simulink model "Test_T_Matrix_VSC"  (R2024a)
settings: Solver=ode2  StartTime=0.0  StopTime=T_end  RelTol=1e-3  EnableMultiTasking=on
values from neighbouring files (symbols this model uses):
  Ts = 5e-6    (= 5e-06)    [Generate_T_Matrix.m]    (also in Test_T_Matrix.m)
undefined symbols (not defined in the file or in its folder): level
libraries: spsabctodq0Lib x5, slpidlib x4, powerlib_extras x3, spsThreePhaseVIMeasurementLib x3, spsThreePhaseSeriesRLCBranchLib x2, simulink_extras x2, spsThreePhaseProgrammableVoltageSourceLib x1, spsGroundLib x1, spsThreePhaseFaultLib x1, spsDCVoltageSourceLib x1, spsUniversalBridgeLib x1, spsdq0toabcLib x1
settings Model: Creator=GAO_CX  LastModifiedBy=GAO_CX
settings DataIOCC: SaveOutput=off  SignalLogging=off  DSMLogging=off  SaveTime=off  ReturnWorkspaceOutputs=off

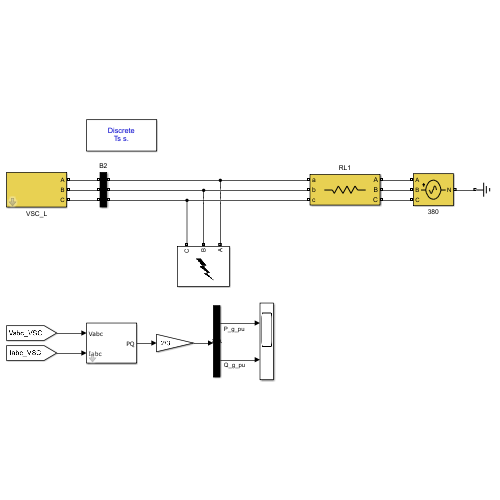
[thumbnail: Simulink's stored preview of the top-level diagram]
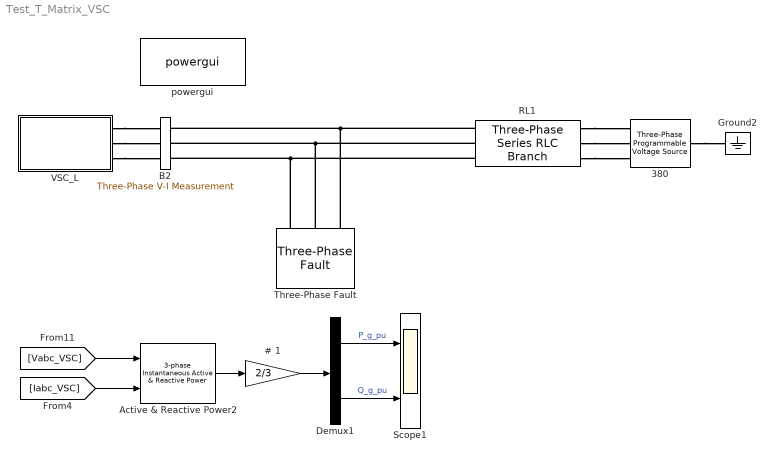
== system Test_T_Matrix_VSC ==
  # 1 : Gain  Gain=2/3  SaturateOnIntegerOverflow=on  OutDataTypeStr=Inherit: Same as input  ParamDataTypeStr=Inherit: Same as input
  380 : spsThreePhaseProgrammableVoltageSourceLib/Three-Phase Programmable Voltage Source  PositiveSequence=[380 0 50]  VariationEntity=None  VariationType=Step  VariationTypeAlt=Step  VariationStep=0.2  VariationRate=10  VariationMagnitude=0.3  VariationFrequency=2  VariationTiming=[20 20.05]  VariationPhaseA=off  Amplitudes=[1 0.5 1]  TimeValues=[0 20 20.3]  HarmonicGeneration=off  HarmonicA=[1 -0.1 0 2]  HarmonicB=[2 0.15 35 2]*0  Timing="[0.1  2]"  BusType=PQ  Pref=0  Qref=0  Qmin=-inf  Qmax=inf
  Active & Reactive Power2 : powerlib_extras/Measurements/3-phase  Instantaneous  Active & Reactive Power
  B2 : spsThreePhaseVIMeasurementLib/Three-Phase V-I Measurement  VoltageMeasurement=phase-to-ground  SetLabelV=on  LabelV=Vabc_VSC  Vpu=on  VpuLL=off  CurrentMeasurement=yes  SetLabelI=on  LabelI=Iabc_VSC  Ipu=on  Pbase=1e6  Vbase=380  OutputType=Complex  PhasorSimulation=off  PSBequivalent=0
  Demux1 : Demux  Outputs=2
      settings: DisplayOption=none
  Ground2 : spsGroundLib/Ground  LConnTagsString=a
  RL1 : spsThreePhaseSeriesRLCBranchLib/Three-Phase Series RLC Branch  LConnTagsString=A|B|C  RConnTagsString=A|B|C  BranchType=R  Resistance=0.01  Inductance=4e-6  Capacitance=1.0  Measurements=None
  Scope1 : Scope  NumInputPorts=2
  Three-Phase Fault : spsThreePhaseFaultLib/Three-Phase Fault  InitialStates=0  FaultA=on  FaultB=off  FaultC=off  GroundFault=on  SwitchTimes=[0.1 0.15]  External=off  SwitchStatus=NaN  FaultResistance=1e-6  GroundResistance=1e-9  SnubberResistance=inf  SnubberCapacitance=inf  Measurements=None
  VSC_L : Subsystem  mask{P_rated=1e6, Vac_rated=380, Vdc_rated=1200, f_rated=50, Pref=1.0, Qref=0, Rf1_pu=1e-3, Lf1_pu=0.5, KP_PLL=5, KI_PLL=100, KP_ig=5, KI_ig=10, KP_P=0.2, KI_P=100}
      mask prompts: P_rated "Rated Power (W)"; Vac_rated "Rated AC voltage (V)"; Vdc_rated "Rated DC voltage (V)"; f_rated "Rated grid frequency"; Rf1_pu "Filter resistor Rf1 (pu)"; Lf1_pu "Filter inductor Lf1 (pu)"; KP_PLL "P of PLL"; KI_PLL "I of PLL"; KP_ig "P of current PI  controller"; KI_ig "I of current PI  controller"; KP_P "P of power PI  controller"; KI_P "I of power PI  controller"
      mask init:
      | Z_rated=Vac_rated*Vac_rated/P_rated;
      | % transformer to pu
      | wg_rated=2*pi*f_rated;
      | Lg_rated=Z_rated/wg_rated;
      | Cg_rated=1/Z_rated/wg_rated;
      | 
      | Rf1=Z_rated*Rf1_pu;
      | Lf1=Lg_rated*Lf1_pu;
      mask DialogControl Basic_Parameters Prompt: Basic Parameters
      mask DialogControl GSC Prompt: GSC Parameters
  powergui : spspowerguiLib/powergui  SimulationMode=Discrete  SampleTime=Ts  frequency=50  Iterations=50  frequencyindice=0  Pbase=100e6  ErrMax=1e-4  UnitsV=kV  UnitsW=MW  buscounter=6  FunctionMessages=off  echomessages=off  EnableUseOfTLC=off  CurrentSourceSwitches=off  DisableSnubberDevices=off  DisableRonSwitches=off  DisableVfSwitches=off  DisplayEquations=off  AutomaticDiscreteSolvers=off  SolverType=Tustin  Interpol=off  ExternalGateDelay=off  methode=off  Ts=0  x0status=blocks  SPID=off  SwTol=0  HookPort=off  NonlinearTolerance=1e-4  nMaxIteration=100  ContinueOnMaxIteration=off  RestoreLinks=warning  ResistiveCurrentMeasurement=off  Frange=[0:2:500]  Ylog=off  Xlog=on  ShowGrid=off  save=off  variable=ZData  structure=0  ZoomFFT=on  StartTime=0.0  cycles=1  DisplayStyle=1  fundamental=60  FreqAxis=off  MaxFrequency=1000  frequencyindicesteady=1  RmsSteady=1  display=off
  wires:
  Demux1/1 -> Scope1/1  "P_g_pu"
  Demux1/2 -> Scope1/2  "Q_g_pu"
  Active & Reactive Power2/1 -> # 1/1
  # 1/1 -> Demux1/1
  [Vabc_VSC] -> Active & Reactive Power2/1
  [Iabc_VSC] -> Active & Reactive Power2/2
  connections:
  RL1/RConn2 -- Three-Phase Fault/LConn2 -- B2/RConn2
  VSC_L/LConn3 -- B2/LConn3
  RL1/LConn1 -- 380/RConn1
  380/LConn1 -- Ground2/LConn1
  VSC_L/LConn1 -- B2/LConn1
  RL1/LConn3 -- 380/RConn3
  VSC_L/LConn2 -- B2/LConn2
  RL1/LConn2 -- 380/RConn2
  RL1/RConn3 -- B2/RConn3 -- Three-Phase Fault/LConn3
  RL1/RConn1 -- Three-Phase Fault/LConn1 -- B2/RConn1

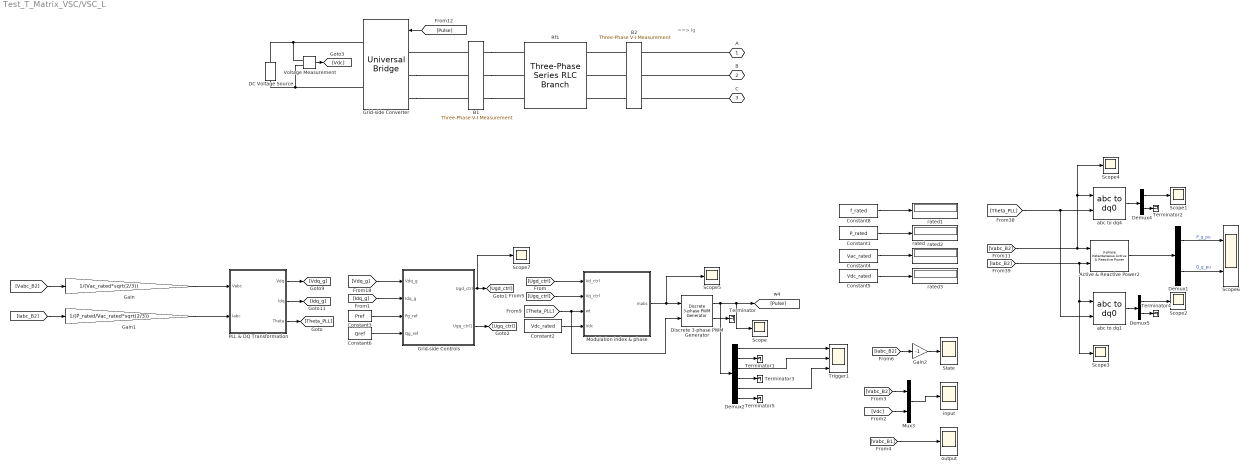
== system Test_T_Matrix_VSC/VSC_L ==
  note: ==> Ig
  Active & Reactive Power2 : powerlib_extras/Measurements/3-phase  Instantaneous  Active & Reactive Power
  B1 : spsThreePhaseVIMeasurementLib/Three-Phase V-I Measurement  VoltageMeasurement=phase-to-ground  SetLabelV=on  LabelV=Vabc_B1  Vpu=off  VpuLL=off  CurrentMeasurement=no  SetLabelI=off  LabelI=Iabc_B1  Ipu=off  Pbase=P_rated  Vbase=Vac_rated  OutputType=Complex  PhasorSimulation=off  PSBequivalent=0
  B2 : spsThreePhaseVIMeasurementLib/Three-Phase V-I Measurement  VoltageMeasurement=phase-to-ground  SetLabelV=on  LabelV=Vabc_B2  Vpu=off  VpuLL=off  CurrentMeasurement=yes  SetLabelI=on  LabelI=Iabc_B2  Ipu=off  Pbase=P_rated  Vbase=Vac_rated  OutputType=Complex  PhasorSimulation=off  PSBequivalent=0
  Constant1 : Constant  Value=P_rated
  Constant2 : Constant  Value=Vdc_rated
  Constant3 : Constant  Value=Pref
  Constant4 : Constant  Value=Vac_rated
  Constant5 : Constant  Value=Vdc_rated
  Constant6 : Constant  Value=Qref
  Constant8 : Constant  Value=f_rated
  DC Voltage Source : spsDCVoltageSourceLib/DC Voltage Source  Amplitude=Vdc_rated  Measurements=None
  Demux1 : Demux  Outputs=2
      settings: DisplayOption=none
  Demux2 : Demux  Outputs=6
      settings: DisplayOption=none
  Demux4 : Demux  Outputs=[2 1]
      settings: DisplayOption=none
  Demux5 : Demux  Outputs=[2 1]
      settings: DisplayOption=none
  Discrete 3-phase PWM Generator : powerlib_extras/Discrete  Control Blocks/Discrete 3-phase PWM Generator  ModulatorType=2-level  ModulatorMode=Synchronized  nF=100  Fc=2700  ModulatingSignals=off  m=0.2  Freq=60  Phase=0  Ts=Ts
  Gain : Gain  Gain=1/(Vac_rated*sqrt(2/3))
  Gain1 : Gain  Gain=1/(P_rated/Vac_rated*sqrt(2/3))
  Gain2 : Gain  Gain=-1
  Grid-side Converter : spsUniversalBridgeLib/Universal Bridge  Arms=3  SnubberResistance=1e6  SnubberCapacitance=inf  Device=IGBT / Diodes  Ron=0.01  Lon=0  ForwardVoltages="[  0  0  ]"  ForwardVoltage=0  GTOparameters=[ 10e-6 , 20e-6 ]  IGBTparameters=[0 , 0]  Measurements=None  Measurements_2=None  converterType=Rectifier
  Grid-side Controls : Subsystem
  "Modulation index & phase " : Subsystem
  Mux3 : Mux  Inputs=2
  PLL & DQ Transformation : Subsystem
  Rf1 : spsThreePhaseSeriesRLCBranchLib/Three-Phase Series RLC Branch  LConnTagsString=A|B|C  RConnTagsString=A|B|C  BranchType=RL  Resistance=Rf1  Inductance=Lf1  Capacitance=1.0  Measurements=None
  Scope{,1..5,7} (7 alike) : Scope
  Scope6 : Scope  NumInputPorts=2
  State : Scope
  Terminator{,1..5} (6 alike) : Terminator
  Trigger1 : Scope  NumInputPorts=3
  Voltage Measurement : spsVoltageMeasurementLib/Voltage Measurement  PhasorSimulation=off  OutputType=Complex  PSBequivalent=0
  abc to dq1 : spsabctodq0Lib/abc to dq0  Alignment=90 degrees behind phase A axis
  abc to dq4 : spsabctodq0Lib/abc to dq0  Alignment=90 degrees behind phase A axis
  input : Scope
  output : Scope
  rated{,1..3} (4 alike) : Display
  A : PMIOPort  Tag=PMCPort  Side=Left
  B : PMIOPort  Tag=PMCPort  Port=2  Side=Left
  C : PMIOPort  Tag=PMCPort  Port=3  Side=Left
  wires:
  PLL & DQ Transformation/3(Theta) -> [Theta_PLL]
  PLL & DQ Transformation/1(Vdq) -> [Vdq_g]
  PLL & DQ Transformation/2(Idq) -> [Idq_g]
  [Vabc_B2] -> Gain/1
  [Iabc_B2] -> Gain1/1
  [Theta_PLL] -> Discrete 3-phase PWM Generator/2, "Modulation index & phase "/3(wt)
  Constant2/1 -> "Modulation index & phase "/4(Vdc)
  [Ugd_ctrl] -> "Modulation index & phase "/1(Vd_ctrl)
  [Ugq_ctrl] -> "Modulation index & phase "/2(Vq_ctrl)
  Grid-side Controls/1(Ugd_ctrl) -> Scope7/1, [Ugd_ctrl]
  Grid-side Controls/2(Ugq_ctrl1) -> [Ugq_ctrl]
  [Vdq_g] -> Grid-side Controls/1(Vdq_g)
  [Idq_g] -> Grid-side Controls/2(Idq_g)
  Constant6/1 -> Grid-side Controls/4(Qg_ref)
  Constant3/1 -> Grid-side Controls/3(Pg_ref)
  [Pulse] -> Grid-side Converter/1
  abc to dq1/1 -> Demux5/1
  Constant5/1 -> rated3/1
  Constant4/1 -> rated/1
  Demux5/1 -> Scope2/1
  [Iabc_B2] -> Scope3/1, abc to dq1/1, Active & Reactive Power2/2
  Demux1/1 -> Scope6/1  "P_g_pu"
  Demux4/1 -> Scope1/1
  [Vabc_B2] -> Scope4/1, abc to dq4/1, Active & Reactive Power2/1
  Constant1/1 -> rated2/1
  [Theta_PLL] -> abc to dq1/2, abc to dq4/2
  Constant8/1 -> rated1/1
  abc to dq4/1 -> Demux4/1
  Active & Reactive Power2/1 -> Demux1/1
  Demux5/2 -> Terminator4/1
  Demux1/2 -> Scope6/2  "Q_g_pu"
  Demux4/2 -> Terminator2/1
  Discrete 3-phase PWM Generator/2 -> Terminator/1
  Discrete 3-phase PWM Generator/1 -> Demux2/1, Scope/1, [Pulse]
  "Modulation index & phase "/1(mabc) -> Scope5/1, Discrete 3-phase PWM Generator/1
  Demux2/1 -> Trigger1/1
  Demux2/2 -> Terminator1/1
  Demux2/3 -> Trigger1/2
  Demux2/5 -> Trigger1/3
  Demux2/4 -> Terminator3/1
  Demux2/6 -> Terminator5/1
  [Iabc_B2] -> Gain2/1
  [Vabc_B1] -> output/1
  Gain/1 -> PLL & DQ Transformation/1(Vabc)
  Gain1/1 -> PLL & DQ Transformation/2(Iabc)
  Voltage Measurement/1 -> [Vdc]
  [Vdc] -> Mux3/2
  [Vabc_B2] -> Mux3/1
  Mux3/1 -> input/1
  Gain2/1 -> State/1
  connections:
  C/RConn1 -- B2/RConn3
  B/RConn1 -- B2/RConn2
  A/RConn1 -- B2/RConn1
  Grid-side Converter/RConn2 -- Voltage Measurement/LConn2 -- DC Voltage Source/LConn1
  Grid-side Converter/RConn1 -- Voltage Measurement/LConn1 -- DC Voltage Source/RConn1
  B2/LConn1 -- Rf1/LConn1
  B2/LConn2 -- Rf1/LConn2
  B2/LConn3 -- Rf1/LConn3
  B1/RConn1 -- Rf1/RConn1
  B1/RConn2 -- Rf1/RConn2
  B1/RConn3 -- Rf1/RConn3
  B1/LConn1 -- Grid-side Converter/LConn1
  Grid-side Converter/LConn2 -- B1/LConn2
  Grid-side Converter/LConn3 -- B1/LConn3

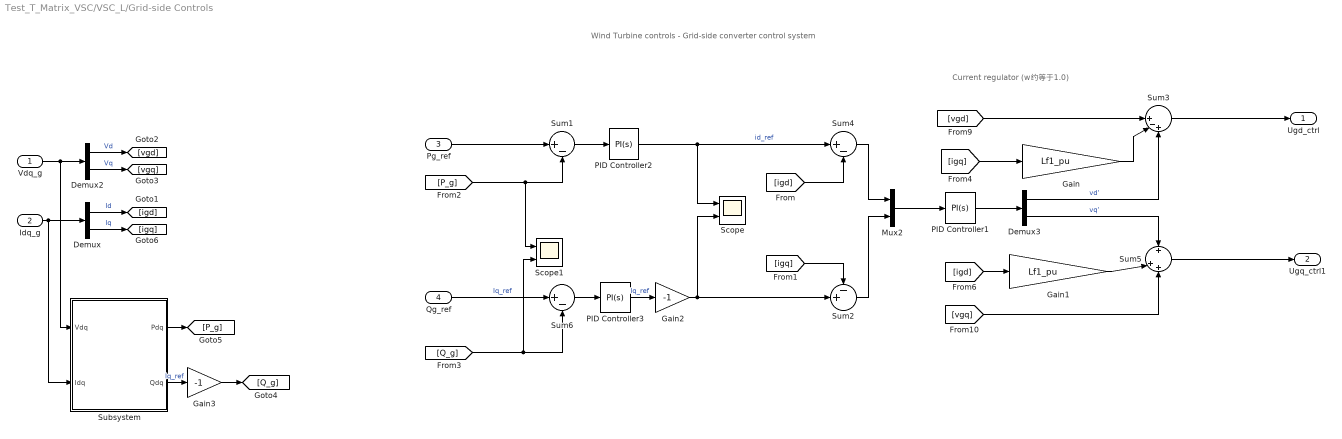
== system Test_T_Matrix_VSC/VSC_L/Grid-side Controls ==
  note: Wind Turbine controls - Grid-side converter control system
  note: Current regulator (w约等于1.0)
  Vdq_g : Inport
  Idq_g : Inport  Port=2
  Pg_ref : Inport  Port=3
  Qg_ref : Inport  Port=4
  Demux : Demux  Outputs=2
      settings: DisplayOption=none
  Demux2 : Demux  Outputs=2
      settings: DisplayOption=none
  Demux3 : Demux  Outputs=2
      settings: DisplayOption=none
  Gain : Gain  Gain=Lf1_pu
  Gain1 : Gain  Gain=Lf1_pu
  Gain2 : Gain  Gain=-1
  Gain3 : Gain  Gain=-1
  Mux2 : Mux  Inputs=2
  PID Controller1 : slpidlib/PID Controller  Controller=PI  Form=Parallel  TimeDomain=Continuous-time  UseExternalTs=off  SampleTime=-1  IntegratorMethod=Forward Euler  FilterMethod=Forward Euler  ControllerParametersSource=internal  P=KP_ig  I=KI_ig  UseKiTs=off  D=0  UseExternalDerivativeSource=off  N=100  UseFilter=on  TunerSelectOption=Transfer Function Based (PID Tuner App)  InitialConditionSource=internal  InitialConditionForIntegrator=0  InitialConditionForFilter=0  DifferentiatorICPrevScaledInput=0  ExternalReset=none  TrackingMode=off  Kt=1  LimitOutput=off  SatLimitsSource=internal  UpperSaturationLimit=5  LowerSaturationLimit=-5  LinearizeAsGain=on  AntiWindupMode=none  Kb=1  LimitIntegrator=off  UpperIntegratorSaturationLimit=inf  LowerIntegratorSaturationLimit=-inf  POutMin=[]  POutMax=[]  IOutMin=[]  IOutMax=[]  DOutMin=[]  DOutMax=[]  NOutMin=[]  NOutMax=[]  SumOutMin=[]  SumOutMax=[]  SaturationOutMin=[]  SaturationOutMax=[]  PParamMin=[]  PParamMax=[]  IParamMin=[]  IParamMax=[]  DParamMin=[]  DParamMax=[]  NParamMin=[]  NParamMax=[]  KbParamMin=[]  KbParamMax=[]  KtParamMin=[]  KtParamMax=[]  KbOutMin=[]  KbOutMax=[]  KtOutMin=[]  KtOutMax=[]  IntegratorOutMin=[]  IntegratorOutMax=[]  FilterOutMin=[]  FilterOutMax=[]  SumI1OutMin=[]  SumI1OutMax=[]  SumI2OutMin=[]  SumI2OutMax=[]  SumI3OutMin=[]  SumI3OutMax=[]  SumI4OutMin=[]  SumI4OutMax=[]  SumDOutMin=[]  SumDOutMax=[]  DifferentiatorOutMin=[]  DifferentiatorOutMax=[]  FilterDiffOutCoefMin=[]  FilterDiffOutCoefMax=[]  ReciprocalOutMin=[]  ReciprocalOutMax=[]  SumDenOutMin=[]  SumDenOutMax=[]  SumNumOutMin=[]  SumNumOutMax=[]  DivideOutMin=[]  DivideOutMax=[]  UdiffTsProdOutMin=[]  UdiffTsProdOutMax=[]  NTsProdOutMin=[]  NTsProdOutMax=[]  UintegralTsProdOutMin=[]  UintegralTsProdOutMax=[]  UngainTsProdOutMin=[]  UngainTsProdOutMax=[]  ClampingZeroOutDataTypeStr=Inherit: Inherit via back propagation  ClampingZeroOutMin=[]  ClampingZeroOutMax=[]  FilterDenConstantOutDataTypeStr=Inherit: Inherit via back propagation  FilterDenConstantOutMin=[]  FilterDenConstantOutMax=[]  PCopyOutDataTypeStr=Inherit: Inherit via back propagation  PCopyOutMin=[]  PCopyOutMax=[]  NCopyOutDataTypeStr=Inherit: Inherit via back propagation  NCopyOutMin=[]  NCopyOutMax=[]  IntegratorContinuousStateAttributes=''  IntegratorStateMustResolveToSignalObject=off  IntegratorRTWStateStorageClass=Auto  FilterContinuousStateAttributes=''  FilterStateMustResolveToSignalObject=off  FilterRTWStateStorageClass=Auto  ParallelPVariant=InternalParameters  IdealPVariant=Disabled  IVariant=InternalParameters  DVariant=Disabled  IntegratorVariant=Continuous  SatVariant=Disabled  AWVariant=Passthrough  PCopyVariant=Disabled  TRVariant=Disabled  FdbkBlocksVariant=Forward  IdealPFdbkVariant=Disabled  SatFdbkVariant=Disabled  DerivativeFilterVariant=Disabled  NVariant=Disabled  NCopyVariant=Disabled_SignalSpec  FilterICVariant=Disabled  IntegratorICVariant=InternalICs  ExternalResetVariant=Disabled  TRSumVariant=Passthrough  SumFdbkVariant=Disabled  SumVariant=Sum_PI  TsampFilterVariant=InternalTs  TsampNgainVariant=Passthrough  TsampIntegralVariant=Disabled_SignalSpec  ExternalSaturationOutDataTypeStr=Inherit: Same as second input  DerivativeSourceVariant=Disabled
  PID Controller2 : slpidlib/PID Controller  Controller=PI  Form=Parallel  TimeDomain=Continuous-time  UseExternalTs=off  SampleTime=-1  IntegratorMethod=Forward Euler  FilterMethod=Forward Euler  ControllerParametersSource=internal  P=KP_P  I=KI_P  UseKiTs=off  D=0  UseExternalDerivativeSource=off  N=100  UseFilter=on  TunerSelectOption=Transfer Function Based (PID Tuner App)  InitialConditionSource=internal  InitialConditionForIntegrator=0  InitialConditionForFilter=0  DifferentiatorICPrevScaledInput=0  ExternalReset=none  TrackingMode=off  Kt=1  LimitOutput=off  SatLimitsSource=internal  UpperSaturationLimit=5  LowerSaturationLimit=-5  LinearizeAsGain=on  AntiWindupMode=none  Kb=1  LimitIntegrator=off  UpperIntegratorSaturationLimit=inf  LowerIntegratorSaturationLimit=-inf  POutMin=[]  POutMax=[]  IOutMin=[]  IOutMax=[]  DOutMin=[]  DOutMax=[]  NOutMin=[]  NOutMax=[]  SumOutMin=[]  SumOutMax=[]  SaturationOutMin=[]  SaturationOutMax=[]  PParamMin=[]  PParamMax=[]  IParamMin=[]  IParamMax=[]  DParamMin=[]  DParamMax=[]  NParamMin=[]  NParamMax=[]  KbParamMin=[]  KbParamMax=[]  KtParamMin=[]  KtParamMax=[]  KbOutMin=[]  KbOutMax=[]  KtOutMin=[]  KtOutMax=[]  IntegratorOutMin=[]  IntegratorOutMax=[]  FilterOutMin=[]  FilterOutMax=[]  SumI1OutMin=[]  SumI1OutMax=[]  SumI2OutMin=[]  SumI2OutMax=[]  SumI3OutMin=[]  SumI3OutMax=[]  SumI4OutMin=[]  SumI4OutMax=[]  SumDOutMin=[]  SumDOutMax=[]  DifferentiatorOutMin=[]  DifferentiatorOutMax=[]  FilterDiffOutCoefMin=[]  FilterDiffOutCoefMax=[]  ReciprocalOutMin=[]  ReciprocalOutMax=[]  SumDenOutMin=[]  SumDenOutMax=[]  SumNumOutMin=[]  SumNumOutMax=[]  DivideOutMin=[]  DivideOutMax=[]  UdiffTsProdOutMin=[]  UdiffTsProdOutMax=[]  NTsProdOutMin=[]  NTsProdOutMax=[]  UintegralTsProdOutMin=[]  UintegralTsProdOutMax=[]  UngainTsProdOutMin=[]  UngainTsProdOutMax=[]  ClampingZeroOutDataTypeStr=Inherit: Inherit via back propagation  ClampingZeroOutMin=[]  ClampingZeroOutMax=[]  FilterDenConstantOutDataTypeStr=Inherit: Inherit via back propagation  FilterDenConstantOutMin=[]  FilterDenConstantOutMax=[]  PCopyOutDataTypeStr=Inherit: Inherit via back propagation  PCopyOutMin=[]  PCopyOutMax=[]  NCopyOutDataTypeStr=Inherit: Inherit via back propagation  NCopyOutMin=[]  NCopyOutMax=[]  IntegratorContinuousStateAttributes=''  IntegratorStateMustResolveToSignalObject=off  IntegratorRTWStateStorageClass=Auto  FilterContinuousStateAttributes=''  FilterStateMustResolveToSignalObject=off  FilterRTWStateStorageClass=Auto  ParallelPVariant=InternalParameters  IdealPVariant=Disabled  IVariant=InternalParameters  DVariant=Disabled  IntegratorVariant=Continuous  SatVariant=Disabled  AWVariant=Passthrough  PCopyVariant=Disabled  TRVariant=Disabled  FdbkBlocksVariant=Forward  IdealPFdbkVariant=Disabled  SatFdbkVariant=Disabled  DerivativeFilterVariant=Disabled  NVariant=Disabled  NCopyVariant=Disabled_SignalSpec  FilterICVariant=Disabled  IntegratorICVariant=InternalICs  ExternalResetVariant=Disabled  TRSumVariant=Passthrough  SumFdbkVariant=Disabled  SumVariant=Sum_PI  TsampFilterVariant=InternalTs  TsampNgainVariant=Passthrough  TsampIntegralVariant=Disabled_SignalSpec  ExternalSaturationOutDataTypeStr=Inherit: Same as second input  DerivativeSourceVariant=Disabled
  PID Controller3 : slpidlib/PID Controller  Controller=PI  Form=Parallel  TimeDomain=Continuous-time  UseExternalTs=off  SampleTime=-1  IntegratorMethod=Forward Euler  FilterMethod=Forward Euler  ControllerParametersSource=internal  P=KP_P  I=KI_P  UseKiTs=off  D=0  UseExternalDerivativeSource=off  N=100  UseFilter=on  TunerSelectOption=Transfer Function Based (PID Tuner App)  InitialConditionSource=internal  InitialConditionForIntegrator=0  InitialConditionForFilter=0  DifferentiatorICPrevScaledInput=0  ExternalReset=none  TrackingMode=off  Kt=1  LimitOutput=off  SatLimitsSource=internal  UpperSaturationLimit=5  LowerSaturationLimit=-5  LinearizeAsGain=on  AntiWindupMode=none  Kb=1  LimitIntegrator=off  UpperIntegratorSaturationLimit=inf  LowerIntegratorSaturationLimit=-inf  POutMin=[]  POutMax=[]  IOutMin=[]  IOutMax=[]  DOutMin=[]  DOutMax=[]  NOutMin=[]  NOutMax=[]  SumOutMin=[]  SumOutMax=[]  SaturationOutMin=[]  SaturationOutMax=[]  PParamMin=[]  PParamMax=[]  IParamMin=[]  IParamMax=[]  DParamMin=[]  DParamMax=[]  NParamMin=[]  NParamMax=[]  KbParamMin=[]  KbParamMax=[]  KtParamMin=[]  KtParamMax=[]  KbOutMin=[]  KbOutMax=[]  KtOutMin=[]  KtOutMax=[]  IntegratorOutMin=[]  IntegratorOutMax=[]  FilterOutMin=[]  FilterOutMax=[]  SumI1OutMin=[]  SumI1OutMax=[]  SumI2OutMin=[]  SumI2OutMax=[]  SumI3OutMin=[]  SumI3OutMax=[]  SumI4OutMin=[]  SumI4OutMax=[]  SumDOutMin=[]  SumDOutMax=[]  DifferentiatorOutMin=[]  DifferentiatorOutMax=[]  FilterDiffOutCoefMin=[]  FilterDiffOutCoefMax=[]  ReciprocalOutMin=[]  ReciprocalOutMax=[]  SumDenOutMin=[]  SumDenOutMax=[]  SumNumOutMin=[]  SumNumOutMax=[]  DivideOutMin=[]  DivideOutMax=[]  UdiffTsProdOutMin=[]  UdiffTsProdOutMax=[]  NTsProdOutMin=[]  NTsProdOutMax=[]  UintegralTsProdOutMin=[]  UintegralTsProdOutMax=[]  UngainTsProdOutMin=[]  UngainTsProdOutMax=[]  ClampingZeroOutDataTypeStr=Inherit: Inherit via back propagation  ClampingZeroOutMin=[]  ClampingZeroOutMax=[]  FilterDenConstantOutDataTypeStr=Inherit: Inherit via back propagation  FilterDenConstantOutMin=[]  FilterDenConstantOutMax=[]  PCopyOutDataTypeStr=Inherit: Inherit via back propagation  PCopyOutMin=[]  PCopyOutMax=[]  NCopyOutDataTypeStr=Inherit: Inherit via back propagation  NCopyOutMin=[]  NCopyOutMax=[]  IntegratorContinuousStateAttributes=''  IntegratorStateMustResolveToSignalObject=off  IntegratorRTWStateStorageClass=Auto  FilterContinuousStateAttributes=''  FilterStateMustResolveToSignalObject=off  FilterRTWStateStorageClass=Auto  ParallelPVariant=InternalParameters  IdealPVariant=Disabled  IVariant=InternalParameters  DVariant=Disabled  IntegratorVariant=Continuous  SatVariant=Disabled  AWVariant=Passthrough  PCopyVariant=Disabled  TRVariant=Disabled  FdbkBlocksVariant=Forward  IdealPFdbkVariant=Disabled  SatFdbkVariant=Disabled  DerivativeFilterVariant=Disabled  NVariant=Disabled  NCopyVariant=Disabled_SignalSpec  FilterICVariant=Disabled  IntegratorICVariant=InternalICs  ExternalResetVariant=Disabled  TRSumVariant=Passthrough  SumFdbkVariant=Disabled  SumVariant=Sum_PI  TsampFilterVariant=InternalTs  TsampNgainVariant=Passthrough  TsampIntegralVariant=Disabled_SignalSpec  ExternalSaturationOutDataTypeStr=Inherit: Same as second input  DerivativeSourceVariant=Disabled
  Scope : Scope  NumInputPorts=2
  Scope1 : Scope  NumInputPorts=2
  Subsystem : Subsystem
  Sum1 : Sum  Inputs=|+-  InputSameDT=on  SaturateOnIntegerOverflow=on  OutDataTypeStr=Inherit: Same as first input
  Sum2 : Sum  Inputs=-+|  InputSameDT=on  SaturateOnIntegerOverflow=on  OutDataTypeStr=Inherit: Same as first input
  Sum3 : Sum  Inputs=||+-+  InputSameDT=on  SaturateOnIntegerOverflow=on  OutDataTypeStr=Inherit: Same as first input
  Sum4 : Sum  Inputs=|+-  InputSameDT=on  SaturateOnIntegerOverflow=on  OutDataTypeStr=Inherit: Same as first input
  Sum5 : Sum  Inputs=+|++  InputSameDT=on  SaturateOnIntegerOverflow=on  OutDataTypeStr=Inherit: Same as first input
  Sum6 : Sum  Inputs=|+-  InputSameDT=on  SaturateOnIntegerOverflow=on  OutDataTypeStr=Inherit: Same as first input
  Ugd_ctrl : Outport
  Ugq_ctrl1 : Outport  Port=2
  wires:
  Demux3/2 -> Sum5/1  "vq'"
  Sum2/1 -> Mux2/2
  Sum4/1 -> Mux2/1
  Vdq_g/1 -> Subsystem/1(Vdq), Demux2/1
  PID Controller1/1 -> Demux3/1
  Demux/1 -> [igd]  "Id"
  Demux/2 -> [igq]  "Iq"
  [igd] -> Sum4/2
  [igq] -> Sum2/1
  Demux2/1 -> [vgd]  "Vd"
  Demux2/2 -> [vgq]  "Vq"
  [vgd] -> Sum3/1
  PID Controller3/1 -> Gain2/1  "Iq_ref"
  [igq] -> Gain/1
  Demux3/1 -> Sum3/3  "vd'"
  [vgq] -> Sum5/3
  Mux2/1 -> PID Controller1/1
  Gain/1 -> Sum3/2
  [igd] -> Gain1/1
  Gain1/1 -> Sum5/2
  Sum3/1 -> Ugd_ctrl/1
  Sum5/1 -> Ugq_ctrl1/1
  Idq_g/1 -> Subsystem/2(Idq), Demux/1
  PID Controller2/1 -> Scope/1, Sum4/1  "id_ref"
  Pg_ref/1 -> Sum1/1
  Sum1/1 -> PID Controller2/1
  Qg_ref/1 -> Sum6/1  "Iq_ref"
  Sum6/1 -> PID Controller3/1
  Subsystem/1(Pdq) -> [P_g]
  Subsystem/2(Qdq) -> Gain3/1  "Iq_ref"
  Gain2/1 -> Sum2/2, Scope/2
  Gain3/1 -> [Q_g]
  [Q_g] -> Scope1/2, Sum6/2
  [P_g] -> Scope1/1, Sum1/2

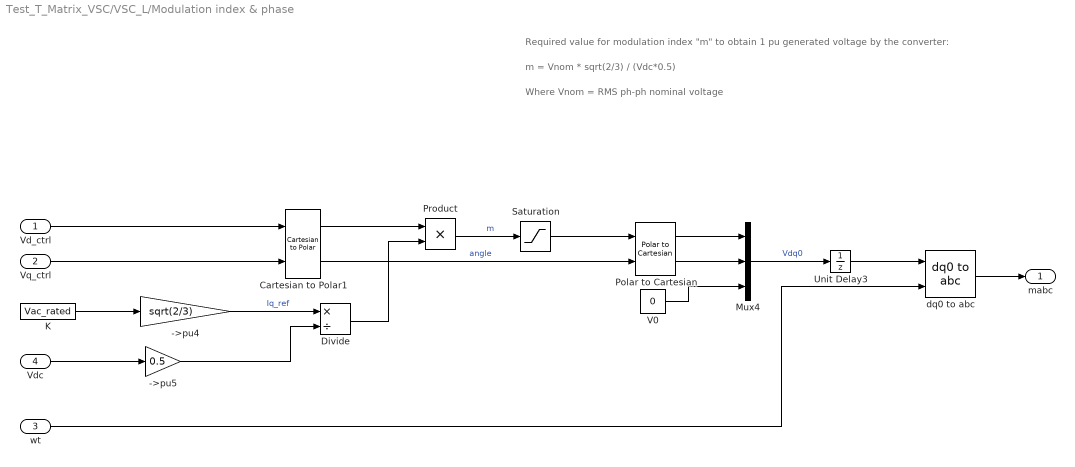
== system Test_T_Matrix_VSC/VSC_L/Modulation index & phase  ==
  note: Where Vnom = RMS ph-ph nominal voltage
  note: m = Vnom * sqrt(2/3) / (Vdc*0.5)
  note: Required value for modulation index "m" to obtain 1 pu generated voltage by the converter:
  Vd_ctrl : Inport
  Vq_ctrl : Inport  Port=2
  wt : Inport  Port=3
  Vdc : Inport  Port=4
  ->pu4 : Gain  Gain=sqrt(2/3)
  ->pu5 : Gain  Gain=0.5
  Cartesian to Polar1 : simulink_extras/Transformations/Cartesian to Polar
  Divide : Product  Inputs=*/
  K : Constant  Value=Vac_rated
  Mux4 : Mux  Inputs=3
  Polar to Cartesian : simulink_extras/Transformations/Polar to Cartesian
  Product : Product
  Saturation : Saturate  UpperLimit=1  LowerLimit=0
  Unit Delay3 : UnitDelay  SampleTime=-1
  V0 : Constant  Value=0
  dq0 to abc : spsdq0toabcLib/dq0 to abc  Alignment=90 degrees behind phase A axis
  mabc : Outport
  wires:
  Cartesian to Polar1/1 -> Product/1
  Mux4/1 -> Unit Delay3/1  "Vdq0"
  Product/1 -> Saturation/1  "m"
  V0/1 -> Mux4/3
  Cartesian to Polar1/2 -> Polar to Cartesian/2  "angle"
  Vdc/1 -> ->pu5/1
  dq0 to abc/1 -> mabc/1
  K/1 -> ->pu4/1
  Vq_ctrl/1 -> Cartesian to Polar1/2
  wt/1 -> dq0 to abc/2
  Vd_ctrl/1 -> Cartesian to Polar1/1
  ->pu5/1 -> Divide/2
  ->pu4/1 -> Divide/1  "Iq_ref"
  Divide/1 -> Product/2
  Polar to Cartesian/1 -> Mux4/1
  Polar to Cartesian/2 -> Mux4/2
  Unit Delay3/1 -> dq0 to abc/1
  Saturation/1 -> Polar to Cartesian/1

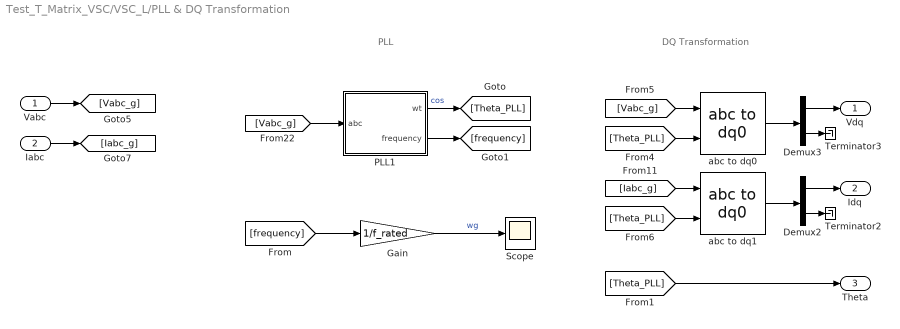
== system Test_T_Matrix_VSC/VSC_L/PLL & DQ Transformation ==
  note: DQ Transformation
  note: PLL
  Vabc : Inport
  Iabc : Inport  Port=2
  Demux2 : Demux  Outputs=[2 1]
      settings: DisplayOption=none
  Demux3 : Demux  Outputs=[2 1]
      settings: DisplayOption=none
  Gain : Gain  Gain=1/f_rated
  PLL1 : Subsystem  mask{KP=KP_PLL, KI=KI_PLL, fbase=f_rated}
      mask DialogControl ParameterGroupVar Prompt: 参数
  Scope : Scope
  Terminator2 : Terminator
  Terminator3 : Terminator
  abc to dq0 : spsabctodq0Lib/abc to dq0  Alignment=90 degrees behind phase A axis
  abc to dq1 : spsabctodq0Lib/abc to dq0  Alignment=90 degrees behind phase A axis
  Vdq : Outport
  Idq : Outport  Port=2
  Theta : Outport  Port=3
  wires:
  Demux2/2 -> Terminator2/1
  abc to dq0/1 -> Demux3/1
  [Theta_PLL] -> abc to dq0/2
  [Theta_PLL] -> abc to dq1/2
  Demux3/2 -> Terminator3/1
  abc to dq1/1 -> Demux2/1
  [Vabc_g] -> PLL1/1(abc)
  [Vabc_g] -> abc to dq0/1
  [Iabc_g] -> abc to dq1/1
  Iabc/1 -> [Iabc_g]
  Vabc/1 -> [Vabc_g]
  [Theta_PLL] -> Theta/1
  PLL1/1(wt) -> [Theta_PLL]  "cos"
  Demux2/1 -> Idq/1
  Demux3/1 -> Vdq/1
  PLL1/2(frequency) -> [frequency]
  [frequency] -> Gain/1
  Gain/1 -> Scope/1  "wg"

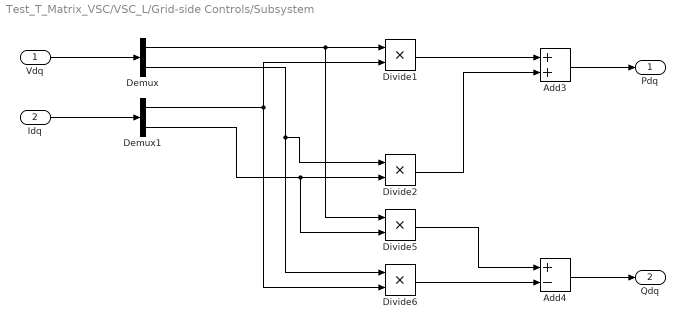
== system Test_T_Matrix_VSC/VSC_L/Grid-side Controls/Subsystem ==
  Vdq : Inport
  Idq : Inport  Port=2
  Add3 : Sum
  Add4 : Sum  Inputs=+-
  Demux : Demux  Outputs=2
  Demux1 : Demux  Outputs=2
  Divide{1..2,5..6} (4 alike) : Product  Inputs=**
  Pdq : Outport
  Qdq : Outport  Port=2
  wires:
  Demux1/1 -> Divide1/2, Divide6/2
  Demux/2 -> Divide6/1, Divide2/1
  Demux1/2 -> Divide5/2, Divide2/2
  Divide5/1 -> Add4/1
  Divide1/1 -> Add3/1
  Add3/1 -> Pdq/1
  Demux/1 -> Divide5/1, Divide1/1
  Divide6/1 -> Add4/2
  Divide2/1 -> Add3/2
  Add4/1 -> Qdq/1
  Vdq/1 -> Demux/1
  Idq/1 -> Demux1/1

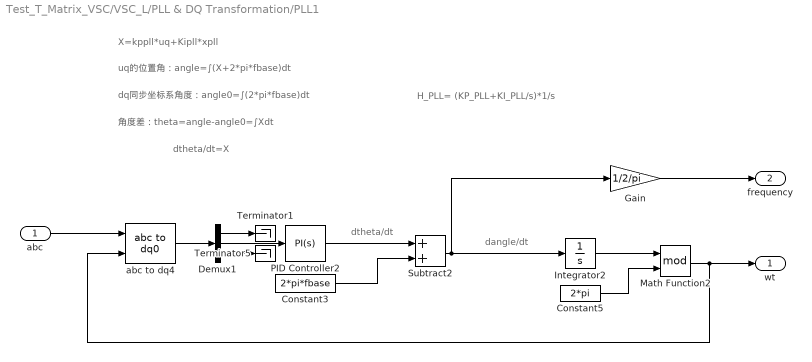
== system Test_T_Matrix_VSC/VSC_L/PLL & DQ Transformation/PLL1 ==
  note: dtheta/dt
  note: uq的位置角：angle=∫(X+2*pi*fbase)dt
  note: dq同步坐标系角度：angle0=∫(2*pi*fbase)dt
  note: 角度差：theta=angle-angle0=∫Xdt
  note: dtheta/dt=X
  note: X=kppll*uq+Kipll*xpll
  note: dangle/dt
  note: H_PLL= (KP_PLL+KI_PLL/s)*1/s
  abc : Inport
  Constant3 : Constant  Value=2*pi*fbase
  Constant5 : Constant  Value=2*pi
  Demux1 : Demux  Outputs=3
  Gain : Gain  Gain=1/2/pi
  Integrator2 : Integrator
  Math Function2 : Math  Operator=mod  SignedPower=on
  PID Controller2 : slpidlib/PID Controller  Controller=PI  Form=Parallel  TimeDomain=Continuous-time  UseExternalTs=off  SampleTime=-1  IntegratorMethod=Forward Euler  FilterMethod=Forward Euler  ControllerParametersSource=internal  P=KP  I=KI  UseKiTs=off  D=1  UseExternalDerivativeSource=off  N=10  UseFilter=on  TunerSelectOption=Transfer Function Based (PID Tuner App)  InitialConditionSource=internal  InitialConditionForIntegrator=0  InitialConditionForFilter=0  DifferentiatorICPrevScaledInput=0  ExternalReset=none  TrackingMode=off  Kt=1  LimitOutput=off  SatLimitsSource=internal  UpperSaturationLimit=2  LowerSaturationLimit=-2  LinearizeAsGain=on  AntiWindupMode=clamping  Kb=1  LimitIntegrator=off  UpperIntegratorSaturationLimit=inf  LowerIntegratorSaturationLimit=-inf  POutMin=[]  POutMax=[]  IOutMin=[]  IOutMax=[]  DOutMin=[]  DOutMax=[]  NOutMin=[]  NOutMax=[]  SumOutMin=[]  SumOutMax=[]  SaturationOutMin=[]  SaturationOutMax=[]  PParamMin=[]  PParamMax=[]  IParamMin=[]  IParamMax=[]  DParamMin=[]  DParamMax=[]  NParamMin=[]  NParamMax=[]  KbParamMin=[]  KbParamMax=[]  KtParamMin=[]  KtParamMax=[]  KbOutMin=[]  KbOutMax=[]  KtOutMin=[]  KtOutMax=[]  IntegratorOutMin=[]  IntegratorOutMax=[]  FilterOutMin=[]  FilterOutMax=[]  SumI1OutMin=[]  SumI1OutMax=[]  SumI2OutMin=[]  SumI2OutMax=[]  SumI3OutMin=[]  SumI3OutMax=[]  SumI4OutMin=[]  SumI4OutMax=[]  SumDOutMin=[]  SumDOutMax=[]  DifferentiatorOutMin=[]  DifferentiatorOutMax=[]  FilterDiffOutCoefMin=[]  FilterDiffOutCoefMax=[]  ReciprocalOutMin=[]  ReciprocalOutMax=[]  SumDenOutMin=[]  SumDenOutMax=[]  SumNumOutMin=[]  SumNumOutMax=[]  DivideOutMin=[]  DivideOutMax=[]  UdiffTsProdOutMin=[]  UdiffTsProdOutMax=[]  NTsProdOutMin=[]  NTsProdOutMax=[]  UintegralTsProdOutMin=[]  UintegralTsProdOutMax=[]  UngainTsProdOutMin=[]  UngainTsProdOutMax=[]  ClampingZeroOutDataTypeStr=Inherit: Inherit via back propagation  ClampingZeroOutMin=[]  ClampingZeroOutMax=[]  FilterDenConstantOutDataTypeStr=Inherit: Inherit via back propagation  FilterDenConstantOutMin=[]  FilterDenConstantOutMax=[]  PCopyOutDataTypeStr=Inherit: Inherit via back propagation  PCopyOutMin=[]  PCopyOutMax=[]  NCopyOutDataTypeStr=Inherit: Inherit via back propagation  NCopyOutMin=[]  NCopyOutMax=[]  IntegratorContinuousStateAttributes=''  IntegratorStateMustResolveToSignalObject=off  IntegratorRTWStateStorageClass=Auto  FilterContinuousStateAttributes=''  FilterStateMustResolveToSignalObject=off  FilterRTWStateStorageClass=Auto  ParallelPVariant=InternalParameters  IdealPVariant=Disabled  IVariant=InternalParameters  DVariant=Disabled  IntegratorVariant=Continuous  SatVariant=Disabled  AWVariant=Passthrough  PCopyVariant=Disabled  TRVariant=Disabled  FdbkBlocksVariant=Forward  IdealPFdbkVariant=Disabled  SatFdbkVariant=Disabled  DerivativeFilterVariant=Disabled  NVariant=Disabled  NCopyVariant=Disabled_SignalSpec  FilterICVariant=Disabled  IntegratorICVariant=InternalICs  ExternalResetVariant=Disabled  TRSumVariant=Passthrough  SumFdbkVariant=Disabled  SumVariant=Sum_PI  TsampFilterVariant=InternalTs  TsampNgainVariant=Passthrough  TsampIntegralVariant=Disabled_SignalSpec  ExternalSaturationOutDataTypeStr=Inherit: Same as second input  DerivativeSourceVariant=Disabled
  Subtract2 : Sum
  Terminator1 : Terminator
  Terminator5 : Terminator
  abc to dq4 : spsabctodq0Lib/abc to dq0  Alignment=90 degrees behind phase A axis
  wt : Outport
  frequency : Outport  Port=2
  wires:
  Math Function2/1 -> wt/1, abc to dq4/2
  Demux1/3 -> Terminator5/1
  PID Controller2/1 -> Subtract2/1
  Constant5/1 -> Math Function2/2
  Constant3/1 -> Subtract2/2
  Integrator2/1 -> Math Function2/1
  abc to dq4/1 -> Demux1/1
  Demux1/1 -> Terminator1/1
  abc/1 -> abc to dq4/1
  Demux1/2 -> PID Controller2/1
  Subtract2/1 -> Gain/1, Integrator2/1
  Gain/1 -> frequency/1
